simulink model "ex8_1"  (R2015a)
settings: Solver=ode23  SolverMode=SingleTasking  StartTime=0.0  StopTime=.2  MaxStep=1e-4  RelTol=1e-4
libraries: powerlib_meascontrol x1, powerlib x1
settings Model: CovMetricSettings=dwe  CovHtmlReporting=off  covSaveCumulativeToWorkspaceVar=off  CovSaveSingleToWorkspaceVar=off  CovExternalEMLEnable=on  Creator=Omid  LastModifiedBy=Omid
settings DataIOCC: LimitDataPoints=off  SaveFormat=Dataset  ReturnWorkspaceOutputs=on
settings DebuggingCC: UnconnectedInputMsg=none  UnconnectedOutputMsg=none  UnconnectedLineMsg=none  SFUnexpectedBacktrackingDiag=error  SFNoUnconditionalDefaultTransitionDiag=error
settings HardwareCC: ProdBitPerPointer=64  ProdLargestAtomicFloat=Float  ProdIntDivRoundTo=Zero  ProdEndianess=LittleEndian  ProdHWDeviceType=Specified
settings ModelReferenceCC: PropagateSignalLabelsOutOfModel=on
settings SFSimCC: SimUseLocalCustomCode=on
settings RTWCC: RTWUseLocalCustomCode=on
settings GRTTargetCC: TargetLangStandard=C99 (ISO)
settings ConfigurationSet: Description=Simscape Multibody

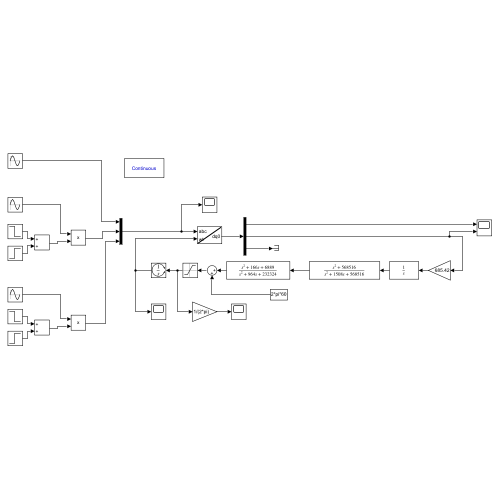
[thumbnail: Simulink's stored preview of the top-level diagram]
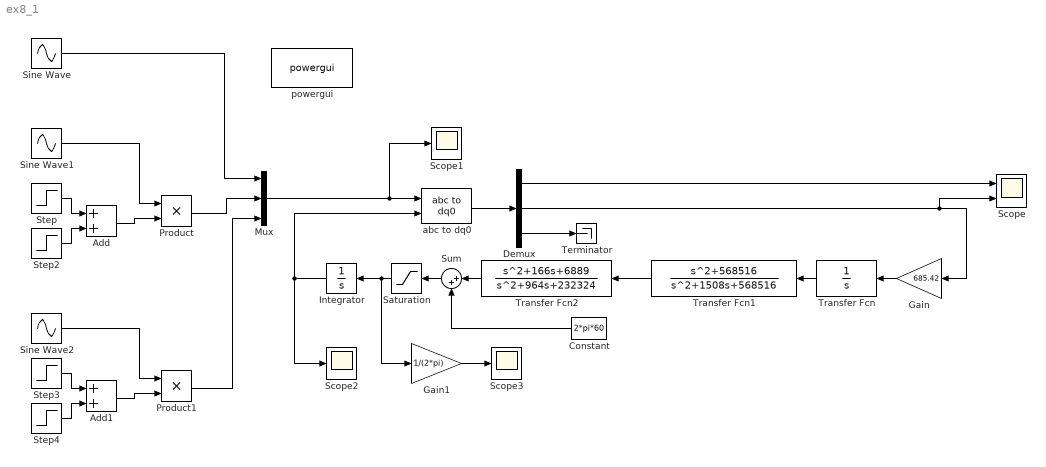
== system ex8_1 ==
  Add : Sum
  Add1 : Sum
  Constant : Constant  Value=2*pi*60
  Demux : Demux  Outputs=3
  Gain : Gain  Gain=685.42
  Gain1 : Gain  Gain=1/(2*pi)
  Integrator : Integrator  WrapState=on  WrappedStateUpperValue=pi*2  WrappedStateLowerValue=0
  Mux : Mux  Inputs=3
  Product : Product
  Product1 : Product
  Saturation : Saturate  UpperLimit=2*pi*75  LowerLimit=2*pi*55
  Scope : Scope  NumInputPorts=2
      settings: TimeRange=auto  MaxDataPoints=5000  SaveToWorkspace=off  SaveName=ScopeData  YMin=-99.35814~-5  YMax=454.60738~5  SampleTime=-1
  Scope1 : Scope
      settings: TimeRange=auto  MaxDataPoints=5000  SaveToWorkspace=off  YMin=-488.64281  YMax=488.64281  SampleTime=-1
  Scope2 : Scope
      settings: TimeRange=auto  MaxDataPoints=5000  SaveToWorkspace=off  SaveName=ScopeData2  YMin=-0.78454  YMax=7.0609  SampleTime=-1
  Scope3 : Scope
      settings: TimeRange=auto  MaxDataPoints=5000  SaveToWorkspace=off  YMin=58.20513  YMax=61.85207  SampleTime=-1
  Sine Wave : Sin  Amplitude=391  Frequency=2*pi*60  Phase=pi/2  SampleTime=0
  Sine Wave1 : Sin  Amplitude=391  Frequency=2*pi*60  Phase=-pi/6  SampleTime=0
  Sine Wave2 : Sin  Amplitude=391  Frequency=2*pi*60  Phase=-5*pi/6  SampleTime=0
  Step : Step  Time=0.05  Before=1  After=0.665  SampleTime=0
  Step2 : Step  Time=0.15  After=0.356  SampleTime=0
  Step3 : Step  Time=0.05  Before=1  After=0.665  SampleTime=0
  Step4 : Step  Time=0.15  After=0.356  SampleTime=0
  Sum : Sum  Inputs=|++
  Terminator : Terminator
  Transfer Fcn : TransferFcn  Denominator=[1 0]
  Transfer Fcn1 : TransferFcn  Numerator=[1 0 568516]  Denominator=[1 1508 568516]
  Transfer Fcn2 : TransferFcn  Numerator=[1 166 6889]  Denominator=[1 964 232324]
  abc to dq0 : powerlib_meascontrol/Transformations/abc to dq0  Alignment=Aligned with phase A axis
  powergui : powerlib/powergui  Priority=1  SimulationMode=Continuous  SampleTime=50e-6  frequency=60  Iterations=50  frequencyindice=60  Pbase=100e6  ErrMax=1e-4  UnitsV=kV  UnitsW=MW  buscounter=0  FunctionMessages=off  echomessages=off  EnableUseOfTLC=off  CurrentSourceSwitches=off  DisableSnubberDevices=off  DisableRonSwitches=off  DisableVfSwitches=off  DisplayEquations=off  AutomaticDiscreteSolvers=off  SolverType=Tustin/Backward Euler (TBE)  Interpol=off  ExternalGateDelay=off  methode=off  Ts=100  x0status=blocks  SPID=on  SwTol=0  HookPort=off  NonlinearTolerance=1e-4  nMaxIteration=100  ContinueOnMaxIteration=off  RestoreLinks=warning  ResistiveCurrentMeasurement=off  Frange=[0:2:500]  Ylog=off  Xlog=on  ShowGrid=off  save=off  variable=ZData  structure=0  ZoomFFT=off  StartTime=0.0  cycles=1  DisplayStyle=1  fundamental=60  FreqAxis=off  MaxFrequency=1000  frequencyindicesteady=1  RmsSteady=1  display=off
  wires:
  Sine Wave/1 -> Mux/1
  Sine Wave2/1 -> Product1/1
  Sine Wave1/1 -> Product/1
  abc to dq0/1 -> Demux/1
  Demux/3 -> Terminator/1
  Demux/1 -> Scope/1
  Demux/2 -> Scope/2, Gain/1
  Integrator/1 -> Scope2/1, abc to dq0/2
  Saturation/1 -> Gain1/1, Integrator/1
  Mux/1 -> Scope1/1, abc to dq0/1
  Transfer Fcn2/1 -> Sum/1
  Sum/1 -> Saturation/1
  Constant/1 -> Sum/2
  Gain1/1 -> Scope3/1
  Transfer Fcn1/1 -> Transfer Fcn2/1
  Transfer Fcn/1 -> Transfer Fcn1/1
  Gain/1 -> Transfer Fcn/1
  Step/1 -> Add/1
  Step2/1 -> Add/2
  Add/1 -> Product/2
  Product/1 -> Mux/2
  Step3/1 -> Add1/1
  Step4/1 -> Add1/2
  Add1/1 -> Product1/2
  Product1/1 -> Mux/3
